simulink model "Orientation_org"  (Simulink 10.0)
settings: Solver=FixedStepDiscrete  StartTime=0.0  StopTime=inf  FixedStep=1e-4  RelTol=1e-3  EnableMultiTasking=on
undefined symbols (not defined in the file): CR, serial
libraries: instrumentlib x4, aerolibanimutils x1, aerolibanim x1, sharedtransform x1
settings Model: Creator=Jorg Angelov  LastModifiedBy=annonymous
settings DataIOCC: LimitDataPoints=on
settings DebuggingCC: UnderspecifiedInitializationDetection=Simplified  MergeDetectMultiDrivingBlocksExec=error  SolverPrmCheckMsg=warning  AllowSymbolicDim=off  SFExecutionAtInitializationDiag=warning
settings GRTTargetCC: GeneratePreprocessorConditionals=Disable all  CombineOutputUpdateFcns=on  GRTInterface=off
settings ConfigComp: CovExternalEMLEnable=off  CovSFcnEnable=off

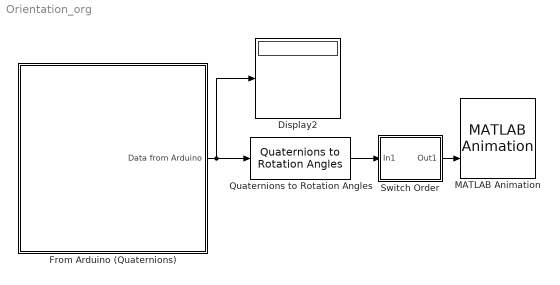
== system Orientation_org ==
  Display2 : Display
  From Arduino (Quaternions) : Subsystem
  MATLAB Animation : aerolibanim/MATLAB Animation  Tag=Matlab Animation 6 DOF  Vehicles=1  Geometries='astredwedge.mat'  BoundingBoxCoordinates=[-50,50,-50,50,-50,50]  CameraOffset=[-150,0,0]  CameraViewAngle=3  SampleTime=-1  FigurePosition=[2,42,798,801]
      settings: SourceProductName=Aerospace Blockset  SourceProductBaseCode=AE
  Quaternions to Rotation Angles : sharedtransform/Quaternions to Rotation Angles  rotationOrder=ZYX  aMode=aMode
      settings: SourceProductBaseCode=AE
  Switch Order : Subsystem  TreatAsAtomicUnit=on
  wires:
  Quaternions to Rotation Angles/1 -> Switch Order/1(In1)
  From Arduino (Quaternions)/1(Data from Arduino) -> Quaternions to Rotation Angles/1, Display2/1
  Switch Order/1(Out1) -> MATLAB Animation/2

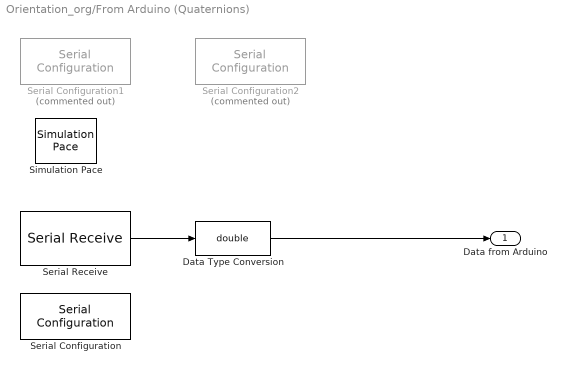
== system Orientation_org/From Arduino (Quaternions) ==
  Data Type Conversion : DataTypeConversion  OutDataTypeStr=double
  Serial Configuration : instrumentlib/Serial Configuration  Priority=-200000  ComPortMenu=<Please select a port...>  ComPort=COM3  ObjConstructor=serial('COM3');  BaudRate=115200  DataBits=8  Parity=none  StopBits=1  FlowControl=none  Timeout=10  ByteOrder=LittleEndian
  Serial Configuration1 : instrumentlib/Serial Configuration  Priority=-200000  Commented=on  ComPortMenu=<Please select a port...>  ComPort=COM5  ObjConstructor=serial('COM5');  BaudRate=115200  DataBits=8  Parity=none  StopBits=1  FlowControl=none  Timeout=10  ByteOrder=LittleEndian
  Serial Configuration2 : instrumentlib/Serial Configuration  Priority=-200000  Commented=on  ComPortMenu=<Please select a port...>  ComPort=COM4  ObjConstructor=serial('COM4');  BaudRate=115200  DataBits=8  Parity=none  StopBits=1  FlowControl=none  Timeout=10  ByteOrder=LittleEndian
  Serial Receive : instrumentlib/Serial Receive  ComPortMenu=COM3  ComPort=COM3  ObjConstructor=serial('COM3');  Header=H  Terminator=CR ('\r')  DataSize=4  DataType=single  EnableBlockingMode=on  ActionDataUnavailable=Output last received value  CustomValue=[1,0,0,0]  SampleTime=0.005
  Simulation Pace : aerolibanimutils/Simulation Pace  SimulationPace=1  SleepMode=MATLAB Thread  OutputPaceError=off  SampleTime=-1
      settings: AttributesFormatString=%<SimulationPace> sec/sec
  Data from Arduino : Outport
  wires:
  Serial Receive/1 -> Data Type Conversion/1
  Data Type Conversion/1 -> Data from Arduino/1

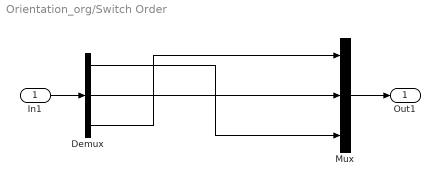
== system Orientation_org/Switch Order ==
  In1 : Inport
  Demux : Demux  Outputs=3
  Mux : Mux  Inputs=3
  Out1 : Outport
  wires:
  In1/1 -> Demux/1
  Demux/1 -> Mux/3
  Demux/3 -> Mux/1
  Demux/2 -> Mux/2
  Mux/1 -> Out1/1
